simulink model "sltestTestSequenceDebouncerExample"  (R2017a)
settings: Solver=ode3  StartTime=0.0  StopTime=50  FixedStep=0.01  RelTol=1e-3  AbsTol=1e-6
model workspace (MAT data in the model file):
  Iei = 0.0219914882836
  converter_data = [0  137.465208994  2.232; 0.1  137.065019157  2.075; 0.2  135.864449646  1.975; 0.3  135.664354728  1.846; 0.4  137.565256453  1.72; 0.5  140.366585312  1.564; 0.6  145.268910814  1.409; 0.7  152.872517717  1.254; 0.8  162.9773111  1.096; 0.81  164.27792807  1.08; 0.82  166.178829795  1.061; 0.83  167.979684062  1.043; 0.84  170.080680706  1.028; 0.85  172.781962105  1.012; 0.86  175.383196045  1.002; 0.87  179.585189333  1.002; 0.88  183.587087703  1.001; 0.89  189.890077635  0.998; 0.9  197.693779455  0.999; 0.92  215.902417037  1.001; 0.94  244.515990379  1.002]
  downtab = [0  5  20  35; 0  5  20  35; 0  5  25  40; 0  5  30  50; 0  30  50  80; 0  30  50  80]
  downth = [0; 5; 40; 50; 90; 100]
  emap = [-40  -44  -49  -53  -57  -61  -65  -70  -74  -78  -82; 215  117  85  66  44  29  10  -2  -13  -22  -32; 245  208  178  148  122  104  85  66  48  33  18; 264  260  241  219  193  167  152  133  119  96  85; 264  279  282  275  260  238  223  208  189  171  152; 267  290  293  297  290  275  260  256  234  212  193; 267  297  305  305  305  301  293  282  267  249  226; 267  301  308  312  319  323  319  316  297  279  253; 267  301  312  319  327  327  327  327  312  293  267; 267  301  312  319  327  334  334  334  319  305  275]
  nevec = [800 1200 1600 2000 2400 2800 3200 3600 4000 4400 4800]
  p0 = 0.07934
  p1 = 0.07934
  thvec = [0; 20; 30; 40; 50; 60; 70; 80; 90; 100]
  uptab = [10  30  50  1000000; 10  30  50  1000000; 15  30  50  1000000; 23  41  60  1000000; 40  70  100  1000000; 40  70  100  1000000]
  upth = [0; 25; 35; 50; 90; 100]
  vehicledata = [3.23; 40; 0.3; 1; 50; 0]
Description:
  | Modeling and testing a simple debouncer using the Test Sequence block
settings Model: ExtModeTrigMode=oneshot  ExtModeArmWhenConnect=off  ExtModeAutoUpdateStatusClock=off  Creator=The MathWorks, Inc.  LastModifiedBy=The MathWorks, Inc.
settings DataIOCC: SaveFormat=Array  SaveOutput=off  SaveTime=off  SignalLoggingName=sigsOut
settings OptimizationCC: BlockReduction=off  BooleanDataType=off  ExpressionDepthLimit=2147483647  InitFltsAndDblsToZero=on  EfficientMapNaN2IntZero=off  LifeSpan=inf
settings DebuggingCC: SaveWithParameterizedLinksMsg=none  UnderspecifiedInitializationDetection=Classic  MergeDetectMultiDrivingBlocksExec=none  CheckExecutionContextPreStartOutputMsg=on  CheckExecutionContextRuntimeOutputMsg=on  SignalResolutionControl=TryResolveAllWithWarning  MultiTaskDSMMsg=warning  MultiTaskCondExecSysMsg=none  IntegerOverflowMsg=none  FcnCallInpInsideContextMsg=warning  AllowSymbolicDim=off  StateNameClashWarn=warning  SFUnexpectedBacktrackingDiag=warning  SFNoUnconditionalDefaultTransitionDiag=warning  SFExecutionAtInitializationDiag=none  IntegerSaturationMsg=none
settings HardwareCC: ProdBitPerPointer=32  ProdBitPerSizeT=32  ProdBitPerPtrDiffT=32  ProdLargestAtomicFloat=None  ProdIntDivRoundTo=Undefined  ProdEndianess=Unspecified  ProdWordSize=32  ProdHWDeviceType=32-bit Generic  TargetBitPerLong=64  TargetBitPerPointer=64  TargetBitPerSizeT=64  TargetBitPerPtrDiffT=64  TargetLongLongMode=on  TargetIntDivRoundTo=Zero  TargetEndianess=LittleEndian  TargetWordSize=64  TargetHWDeviceType=MATLAB Host  ProdEqTarget=off
settings ModelReferenceCC: PropagateSignalLabelsOutOfModel=off
settings SFSimCC: SFSimEcho=off  SimParseCustomCode=off
settings GRTTargetCC: TargetFcnLib=ansi_tfl_tmw.mat  TargetLangStandard=C89/C90 (ANSI)  GeneratePreprocessorConditionals=Disable all  CombineOutputUpdateFcns=off  GRTInterface=on
settings ConfigComp: CovMetricSettings=dcmtr  CovHtmlReporting=on  CovSaveCumulativeToWorkspaceVar=on  CovSaveSingleToWorkspaceVar=on  CovExternalEMLEnable=off  CovSFcnEnable=off

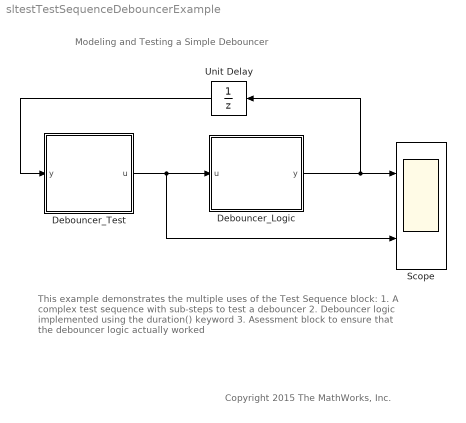
== system sltestTestSequenceDebouncerExample ==
  note: Modeling and Testing a Simple Debouncer
  note: This example demonstrates the multiple uses of the Test Sequence block:
      | 1. A complex test sequence with sub-steps to test a debouncer
      | 2. Debouncer logic implemented using the duration() keyword
      | 3. Asessment block to ensure that the debouncer logic actually worked
  note: Copyright 2015 The MathWorks, Inc.
  Debouncer_Logic : Test Sequence  TreatAsAtomicUnit=on
  Debouncer_Test : Test Sequence  TreatAsAtomicUnit=on
  Scope : Scope  NumInputPorts=2
  Unit Delay : UnitDelay  SampleTime=-1
  wires:
  Debouncer_Test/1(u) -> Scope/2, Debouncer_Logic/1(u)
  Debouncer_Logic/1(y) -> Unit Delay/1, Scope/1
  Unit Delay/1 -> Debouncer_Test/1(y)

== stateflow chart sltestTestSequenceDebouncerExample/Debouncer_Logic ==
  settings: stateMachineType=SIMPLIFIED_MACHINE
  state Off
    % The duration operator is used to implement the debouncing logic.
    % It transitions to the "On" step when the expression u==1
    % stays true for at least 0.5 sec. If u becomes 1 for a period shorter than
    % 0.5 sec, the system remains in this step.
    y = 0;
  state On
    % Transition to the "Off" step when the expression u==0
    % stays true for at least 0.5 sec
    y = 1;
  (default) -> Off
  Off -> On : [duration(u==1) >0.5]
  On -> Off : [duration(u==0)>0.5]
  data: u input; y output

== stateflow chart sltestTestSequenceDebouncerExample/Debouncer_Test ==
  settings: stateMachineType=SIMPLIFIED_MACHINE
  state ALWAYS_OFF
    % Create an input signal to the Debouncing Logic block
    % that toggles fast and slow.
    % Initially, the output is always 0
    u = 0;
  state FAST_TOGGLE_1
    % While in fast_toggle, assert that the value of "y",
    % which is the output of the debouncer does not change.
    % latch(y) returns the value of y when the state is first entered
    % we want the value of y to be the same throughout the execution
    % of this step
    assert(y==latch(y));
    state OFF
      u=0;
    state ON
      u=1;
    (default) -> FAST_TOGGLE_1.OFF
    FAST_TOGGLE_1.OFF -> FAST_TOGGLE_1.ON : [after(0.1,sec)]
    FAST_TOGGLE_1.ON -> FAST_TOGGLE_1.OFF : [after(0.1,sec)]
  state SLOW_TOGGLE_1
    state OFF
      u = 0;
    state ON
      u = 1;
    (default) -> SLOW_TOGGLE_1.OFF
    SLOW_TOGGLE_1.OFF -> SLOW_TOGGLE_1.ON : [after(2,sec)]
    SLOW_TOGGLE_1.ON -> SLOW_TOGGLE_1.OFF : [after(2,sec)]
  state ALWAYS_ON
    u = 1;
  state FAST_TOGGLE_2
    assert(y==latch(y));
    state ON
      u = 1;
    state OFF
      u = 0;
    (default) -> FAST_TOGGLE_2.ON
    FAST_TOGGLE_2.ON -> FAST_TOGGLE_2.OFF : [after(0.1,sec)]
    FAST_TOGGLE_2.OFF -> FAST_TOGGLE_2.ON : [after(0.1,sec)]
  state SLOW_TOGGLE_2
    state ON
      u=1;
    state OFF
      u=0;
    (default) -> SLOW_TOGGLE_2.ON
    SLOW_TOGGLE_2.ON -> SLOW_TOGGLE_2.OFF : [after(2,sec)]
    SLOW_TOGGLE_2.OFF -> SLOW_TOGGLE_2.ON : [after(2,sec)]
  (default) -> ALWAYS_OFF
  ALWAYS_OFF -> FAST_TOGGLE_1 : [after(5,sec)]
  FAST_TOGGLE_1 -> SLOW_TOGGLE_1 : [after(5,sec)]
  SLOW_TOGGLE_1 -> ALWAYS_ON : [after(10,sec)]
  ALWAYS_ON -> FAST_TOGGLE_2 : [after(5,sec)]
  FAST_TOGGLE_2 -> SLOW_TOGGLE_2 : [after(5,sec)]
  data: u output; y input
